simulink library "IFIR"  (R2022b)
settings: Solver=VariableStepAuto  StartTime=0.0  StopTime=10.0  RelTol=1e-3
undefined symbols (not defined in the file or in its folder): MBS
libraries: HandyTextFile x1
settings Model: Creator=ud1041536  LastModifiedBy=jk1043656
settings SolverCC: AlgebraicLoopSolver=TrustRegion
settings DebuggingCC: UnconnectedInputMsg=warning  UnconnectedOutputMsg=warning  UnconnectedLineMsg=warning  SFMachineParentedDataDiag=warning  ArithmeticOperatorsInVariantConditions=warning
settings ModelReferenceCC: EnableRefExpFcnMdlSchedulingChecks=on
settings SFSimCC: CustomCodeUndefinedFunction=UseInterfaceOnly

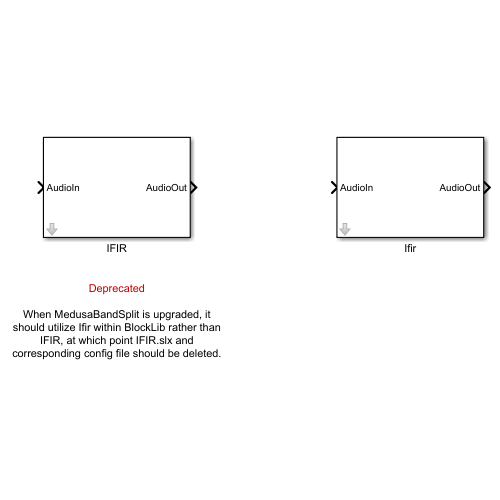
[thumbnail: Simulink's stored preview of the top-level diagram]
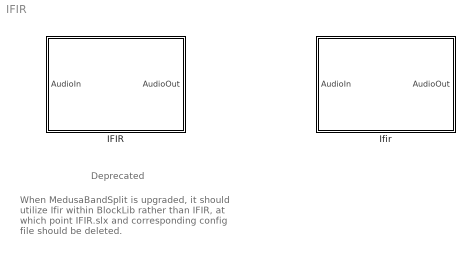
== system IFIR ==
  note: When MedusaBandSplit is upgraded, it should utilize Ifir within BlockLib rather than IFIR, at which point IFIR.slx and corresponding config file should be deleted.
  note: Deprecated
  IFIR : Subsystem  mask(Interpolated FIR){coeffsFlip=MBS.interpolated_filter, I=MBS.D/2, numChannels=2}
      mask prompts: coeffsFlip "Coefficients"; I "Interpolation Factor"; numChannels "Num inputs"
      mask help:
      | An interpolated FIR filter is an FIR filter with a sparse set of coefficients containing I-1 zeros between each point, where I is the interpolation factor.
      |
      | The block supports multiple channels, with each channel sharing the same set of filter coefficients. Users need to specify the non-zero coefficients, the interpolation factor and the number of channels.
      mask init:
      | % Flip the coeffs
      | [~, numCoeffSets] = size(coeffsFlip);
      | ind = 0:numCoeffSets-1;
      | coeffsFlip = flipud(coeffsFlip(:,ind+1));
      | 
      | % Cast decimation factor to int32
      | I = int32(I);
  Ifir : Subsystem  mask(Interpolated FIR){Config=[]}
      mask prompts: Config "IfirConfig"
      mask help:
      | An interpolated FIR filter is an FIR filter with a sparse set of coefficients containing I-1 zeros between each point, where I is the interpolation factor.
      |
      | The block supports multiple channels, with each channel sharing the same set of filter coefficients. Users need to specify the non-zero coefficients, the interpolation factor and the number of channels.
      mask init:
      | blkh=gcbh;
      | Config=BTConfig.Assert(blkh,Config);
      | 
      | Config.Validate();

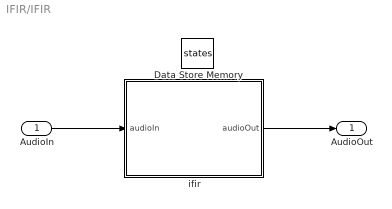
== system IFIR/IFIR ==
  AudioIn : Inport
  Data Store Memory : DataStoreMemory  DataStoreName=states  ReadBeforeWriteMsg=warning  WriteAfterWriteMsg=warning  WriteAfterReadMsg=warning  InitialValue=zeros(size(coeffsFlip,1)*I,numChannels)  ShowAdditionalParam=off  OutDataTypeStr=single
  ifir : MATLAB Function  TreatAsAtomicUnit=on
  AudioOut : Outport  VectorParamsAs1DForOutWhenUnconnected=off
  wires:
  AudioIn/1 -> ifir/1(audioIn)
  ifir/1(audioOut) -> AudioOut/1

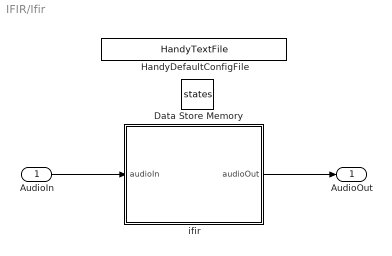
== system IFIR/Ifir ==
  AudioIn : Inport
  Data Store Memory : DataStoreMemory  DataStoreName=states  ReadBeforeWriteMsg=warning  WriteAfterWriteMsg=warning  WriteAfterReadMsg=warning  InitialValue=Config.InitialStates  ShowAdditionalParam=off  OutDataTypeStr=single
  HandyDefaultConfigFile : HandyTextFile/HandyTextFile  TemplateSource=Config  FileSuffix=Init  OpenDialogOnLoad=off  UseThisBlockName=off  AddGrandParentNamePrefix=off  TheDefaultText=|  ShowInLibBrowser=on
      | % $(FILENAME) Setup model parameters for each "Init" callback (e.g. update diagram)
      | sample_rate_in_hertz = 44100;
      | frame_size = 32;
      | sysin_channel_count = 2;
      settings: SourceProductName=Bose Talaria
  ifir : MATLAB Function  TreatAsAtomicUnit=on  mask{FlippedCoefficients=Config.FlippedCoefficients, InterpolationFactor=Config.InterpolationFactor}
  AudioOut : Outport  VectorParamsAs1DForOutWhenUnconnected=off
  wires:
  AudioIn/1 -> ifir/1(audioIn)
  ifir/1(audioOut) -> AudioOut/1

== matlab function IFIR/Ifir/ifir ==
  data: audioIn input; InterpolationFactor parameter; FlippedCoefficients parameter; audioOut output; states data_store_memory
function audioOut = ifir(audioIn, InterpolationFactor, FlippedCoefficients)

% An interpolated FIR filter is an FIR filter with a sparse set of
% coefficients.  That is, the coefficients contain I-1 zeros between
% each point, so the effective length of  filter is len(input_coeffs) * I  
% The function support multiple channels, with each
% channel sharing the same set of filter coefficients.
% 
% p : coefficient set (non-zero coefficients)
% I : interpolation factor, I-1 zeros are inserted between each coefficient
% 
% NOTES: 
% The legacy IFIR block supported coefficient sets.  Currently
% this only supports one coefficient set. 
% The coefficients are stored flipped in time. The unflipped coeffs are
% passed to block mask, and the flipping is done in mask initialization.

% Initialize variables
[frameSize, numChannels] = size(audioIn);
[filterLength, ~] = size(FlippedCoefficients);

frameSize   = uint32(frameSize);
numChannels = uint32(numChannels);
filterLength = int32(filterLength);
activeCoeffSet = coder.const(uint32(zeros(1,numChannels)));

% State is a circular buffer that holds previous stateLen samples, 
% where state_index points to the last/oldest sample in the buffer, which 
% during processing will be overwritten by the current input sample.
global states;

persistent state_index;
if isempty(state_index)
    state_index = int32(0);
end

audioOut = IFIR(audioIn, frameSize, numChannels, states, filterLength, ...
                    state_index, FlippedCoefficients, activeCoeffSet, InterpolationFactor);
                
end

function y = IFIR(audioIn, frameSize, numChannels, states2, filterLength, ...
                    state_index2, FlippedCoefficients, activeCoeffSet, InterpolationFactor)
% If code gen'ing, generate warning if this is not replaced with IFIR.asm
coder.replace('-warnifnoreplacement');

% We have to use a different state buffer and state index than the one 
% passed in.  Matlab value objects are passed by value, not by reference, 
% so the saving of states here does not work.  The state buffer and index 
% are still necessary to pass allocate in the calling function and pass 
% here in order to trigger CRL. This double buffering is annoying, however 
% only happens during simulation, not code generation. (taken from pooliir)
global states;
persistent state_index;
if isempty(state_index)
    state_index = int32(0);
end

y = coder.nullcopy(audioIn);
stateLen = filterLength * InterpolationFactor;

for channel = 1:numChannels
    state = states(:,channel);
    stateIndex = state_index;
    coeffs = FlippedCoefficients(:,activeCoeffSet(channel)+1);
    
    for sample = 1:frameSize
        % overwrite oldest sample with the current input sample
        state(stateIndex+1) = audioIn(sample, channel);
        % go to the oldest sample (previously the 2nd oldest)
        stateIndex = stateIndex + InterpolationFactor; 
        if (stateIndex >= stateLen)
            stateIndex = stateIndex - stateLen;
        end

        accum = single(0);
        for i = 1:filterLength
            accum = accum + (state(stateIndex+1) * coeffs(i));
            stateIndex = stateIndex + InterpolationFactor; % skip zero coefficients
            if (stateIndex >= stateLen)
                    stateIndex = stateIndex - stateLen;
            end
        end
        y(sample, channel) = accum;

        % update stateIndex for next sample
        % because we subtract here state_index type is int32 not uint32
        stateIndex = stateIndex - (InterpolationFactor-1);
        if (stateIndex < 0)
            stateIndex = stateIndex + stateLen;
        end
    end
 
    states(:, channel) = state;
end

state_index = stateIndex;

end

== matlab function IFIR/ifir ==
  data: audioIn input; coeffsFlip parameter; audioOut output; I parameter; states data_store_memory
function audioOut = ifir(audioIn, coeffsFlip, I)

% An interpolated FIR filter is an FIR filter with a sparse set of
% coefficients.  That is, the coefficients contain I-1 zeros between
% each point, so the effective length of  filter is len(input_coeffs) * I  
% The function support multiple channels, with each
% channel sharing the same set of filter coefficients.
% 
% p : coefficient set (non-zero coefficients)
% I : interpolation factor, I-1 zeros are inserted between each coefficient
% 
% NOTES: 
% The legacy IFIR block supported coefficient sets.  Currently
% this only supports one coefficient set. 
% The coefficients are stored flipped in time. The unflipped coeffs are
% passed to block mask, and the flipping is done in mask initialization.

% Initialize variables
[frameSize, numChannels] = size(audioIn);
[filterLength, ~] = size(coeffsFlip);

frameSize   = uint32(frameSize);
numChannels = uint32(numChannels);
filterLength = int32(filterLength);
activeCoeffSet = coder.const(uint32(zeros(1,numChannels)));

% State is a circular buffer that holds previous stateLen samples, 
% where state_index points to the last/oldest sample in the buffer, which 
% during processing will be overwritten by the current input sample.
global states;

persistent state_index;
if isempty(state_index)
    state_index = int32(0);
end

audioOut = IFIR(audioIn, frameSize, numChannels, states, filterLength, ...
                    state_index, coeffsFlip, activeCoeffSet, I);
                
end

function y = IFIR(audioIn, frameSize, numChannels, states2, filterLength, ...
                    state_index2, coeffsFlip, activeCoeffSet, I)
% If code gen'ing, generate warning if this is not replaced with IFIR.asm
coder.replace('-warnifnoreplacement');

% We have to use a different state buffer and state index than the one 
% passed in.  Matlab value objects are passed by value, not by reference, 
% so the saving of states here does not work.  The state buffer and index 
% are still necessary to pass allocate in the calling function and pass 
% here in order to trigger CRL. This double buffering is annoying, however 
% only happens during simulation, not code generation. (taken from pooliir)
global states;
persistent state_index;
if isempty(state_index)
    state_index = int32(0);
end

y = coder.nullcopy(audioIn);
stateLen = filterLength * I;

for channel = 1:numChannels
    state = states(:,channel);
    stateIndex = state_index;
    coeffs = coeffsFlip(:,activeCoeffSet(channel)+1);
    
    for sample = 1:frameSize
        % overwrite oldest sample with the current input sample
        state(stateIndex+1) = audioIn(sample, channel);
        % go to the oldest sample (previously the 2nd oldest)
        stateIndex = stateIndex + I; 
        if (stateIndex >= stateLen)
            stateIndex = stateIndex - stateLen;
        end

        accum = single(0);
        for i = 1:filterLength
            accum = accum + (state(stateIndex+1) * coeffs(i));
            stateIndex = stateIndex + I; % skip zero coefficients
            if (stateIndex >= stateLen)
                    stateIndex = stateIndex - stateLen;
            end
        end
        y(sample, channel) = accum;

        % update stateIndex for next sample
        % because we subtract here state_index type is int32 not uint32
        stateIndex = stateIndex - (I-1);
        if (stateIndex < 0)
            stateIndex = stateIndex + stateLen;
        end
    end
 
    states(:, channel) = state;
end

state_index = stateIndex;

end
